simulink model "MySecondSimulink"  (Simulink 7.6)
settings: Solver=ode45  StartTime=0.0  StopTime=10.0  RelTol=1e-3
settings Model: Creator=Administrator  LastModifiedBy=Administrator

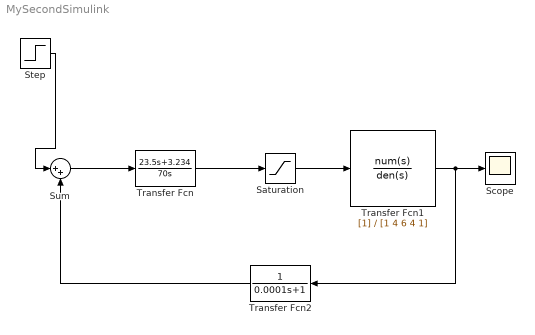
== system MySecondSimulink ==
  Saturation : Saturate
  Scope : Scope
  Step : Step  SampleTime=0
  Sum : Sum  Inputs=|++
  Transfer Fcn : TransferFcn  Numerator=[23.5 3.234]  Denominator=[70 0]
  Transfer Fcn1 : TransferFcn  Denominator=[1 4 6 4 1]
  Transfer Fcn2 : TransferFcn  Denominator=[0.0001 1]
  wires:
  Sum/1 -> Transfer Fcn/1
  Transfer Fcn/1 -> Saturation/1
  Saturation/1 -> Transfer Fcn1/1
  Transfer Fcn1/1 -> Scope/1, Transfer Fcn2/1
  Transfer Fcn2/1 -> Sum/2
  Step/1 -> Sum/1
